simulink model "lectura_respuesta_planta"  (R2021a)
settings: Solver=VariableStepAuto  StartTime=0.0  StopTime=Inf  RelTol=1e-3
libraries: instrumentseriallib x2
settings Model: Creator=Claudio  LastModifiedBy=crist

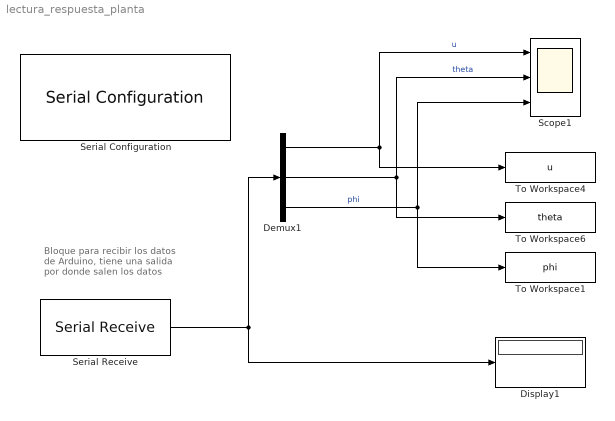
== system lectura_respuesta_planta ==
  note: Bloque para recibir los datos de Arduino, tiene una salida por donde salen los datos
  Demux1 : Demux  Outputs=3
  Display1 : Display
  Scope1 : Scope  NumInputPorts=3
  Serial Configuration : instrumentseriallib/Serial Configuration  Priority=-200000  Port=COM5  ComPort=COM5  BaudRate=115200  DataBits=8  Parity=none  StopBits=1  ByteOrder=big-endian  FlowControl=none  Timeout=10  SimulateUsing=Interpreted execution  BlockInModel=on
  Serial Receive : instrumentseriallib/Serial Receive  Priority=1  Port=COM5  ComPort=COM5  DataType=single  SaveDataType=uint8  ToggleHeader=on  Header=[97 98 99 100]  ToggleTerminator=off  Terminator=<none>  CustomTerminator=[]  ToggleDataSize=on  DataSize=[3 1]  EnableBlockingMode=on  ActionDataUnavailable=Output last received value  ActionWhenDataUnavailable=Output last received value  CustomValue=0  SampleTime=0.01  SimulateUsing=Interpreted execution  BlockInModel=on
  To Workspace1 : ToWorkspace  VariableName=phi  SampleTime=-1
      settings: Save2DSignal=2-D array (concatenate along first dimension)
  To Workspace4 : ToWorkspace  VariableName=u  SampleTime=-1
      settings: Save2DSignal=2-D array (concatenate along first dimension)
  To Workspace6 : ToWorkspace  VariableName=theta  SampleTime=-1
      settings: Save2DSignal=2-D array (concatenate along first dimension)
  wires:
  Demux1/1 -> To Workspace4/1, Scope1/1  "u"
  Demux1/3 -> To Workspace1/1, Scope1/3  "phi"
  Demux1/2 -> To Workspace6/1, Scope1/2  "theta"
  Serial Receive/1 -> Display1/1, Demux1/1
